simulink model "MultiAgentSEIRv1"  (R2019b)
settings: Solver=VariableStepAuto  StartTime=0.0  StopTime=365*2  FixedStep=1/24  RelTol=1e-12
libraries: SEIR_Lib x10
settings Model: Creator=Alex  LastModifiedBy=Alex

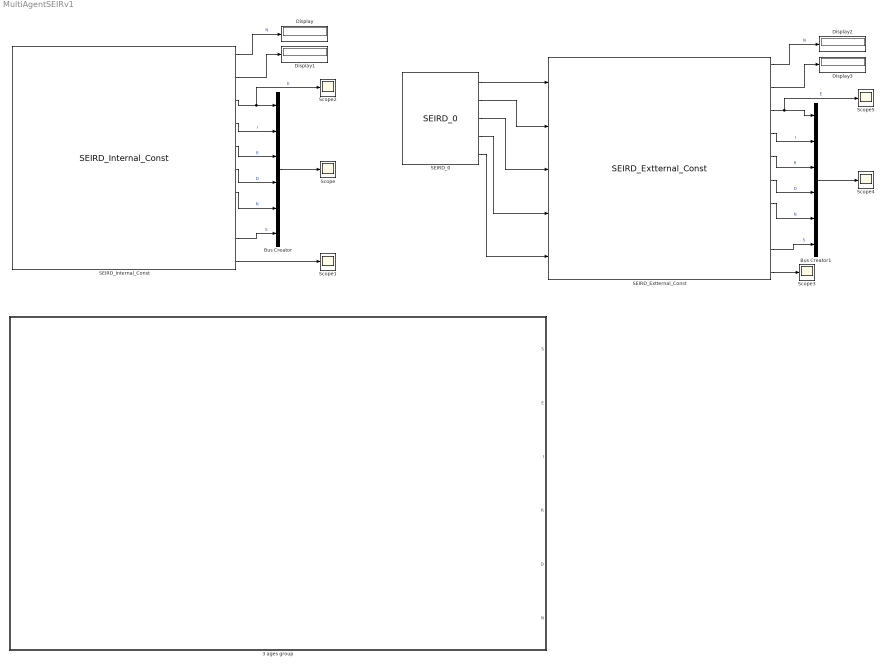
== system MultiAgentSEIRv1 ==
  3 ages group : Subsystem
  Bus Creator : BusCreator  Inputs=6
  Bus Creator1 : BusCreator  Inputs=6
  Display{,1..3} (4 alike) : Display
  SEIRD_0 : SEIR_Lib/SEIRD_0  SystemSampleTime=-1  Latency=0  AutoFrameSizeCalculation=off
  SEIRD_Extternal_Const : SEIR_Lib/SEIRD_Extternal_Const  SystemSampleTime=-1  Latency=0  AutoFrameSizeCalculation=off
      link override alpha1/Random NumberAlpha: Mean=0.1
  SEIRD_Internal_Const : SEIR_Lib/SEIRD_Internal_Const  SystemSampleTime=-1  Latency=0  AutoFrameSizeCalculation=off
      link override alpha1/Random NumberAlpha: Mean=0.1
  Scope{,1..5} (6 alike) : Scope
  wires:
  SEIRD_Internal_Const/3 -> Scope2/1, Bus Creator/1  "E"
  SEIRD_Internal_Const/4 -> Bus Creator/2  "I"
  SEIRD_Internal_Const/5 -> Bus Creator/3  "R"
  SEIRD_Internal_Const/6 -> Bus Creator/4  "D"
  SEIRD_Internal_Const/7 -> Bus Creator/5  "N"
  SEIRD_Internal_Const/9 -> Bus Creator/6  "S"
  Bus Creator/1 -> Scope/1
  SEIRD_Internal_Const/1 -> Display/1  "N"
  SEIRD_Internal_Const/2 -> Display1/1
  SEIRD_Internal_Const/10 -> Scope1/1
  SEIRD_0/1 -> SEIRD_Extternal_Const/1
  SEIRD_0/2 -> SEIRD_Extternal_Const/2
  SEIRD_0/3 -> SEIRD_Extternal_Const/3
  SEIRD_0/4 -> SEIRD_Extternal_Const/4
  SEIRD_0/5 -> SEIRD_Extternal_Const/5
  SEIRD_Extternal_Const/10 -> Scope3/1
  SEIRD_Extternal_Const/2 -> Display3/1
  SEIRD_Extternal_Const/1 -> Display2/1  "N"
  Bus Creator1/1 -> Scope4/1
  SEIRD_Extternal_Const/9 -> Bus Creator1/6  "S"
  SEIRD_Extternal_Const/7 -> Bus Creator1/5  "N"
  SEIRD_Extternal_Const/6 -> Bus Creator1/4  "D"
  SEIRD_Extternal_Const/5 -> Bus Creator1/3  "R"
  SEIRD_Extternal_Const/4 -> Bus Creator1/2  "I"
  SEIRD_Extternal_Const/3 -> Scope5/1, Bus Creator1/1  "E"

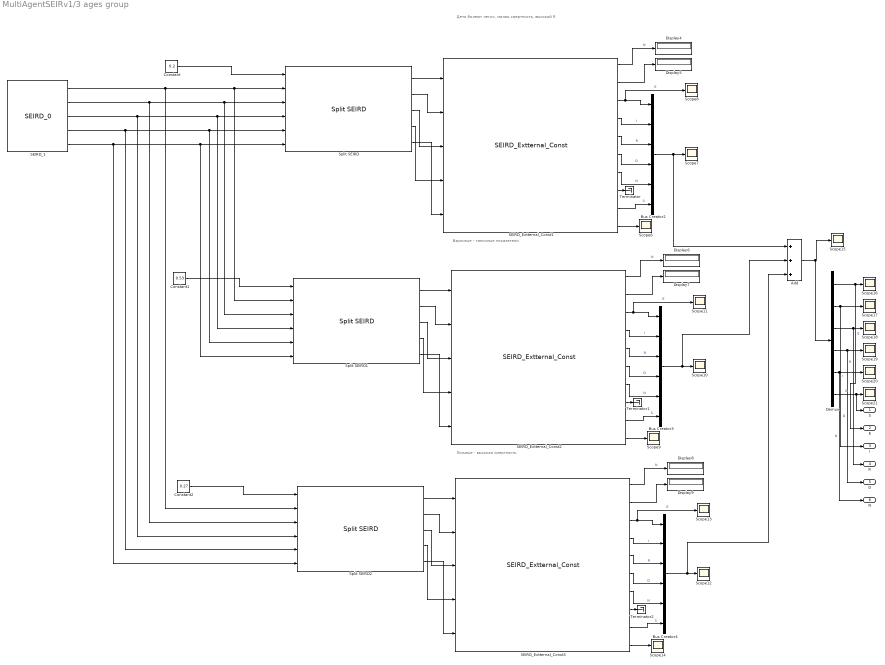
== system MultiAgentSEIRv1/3 ages group ==
  note: Пожиые - высокая смертность
  note: Взрослые - типичные показатели
  note: Дети болеют легко, малая смертность, высокий R
  Add : Sum  Inputs=+++
  Bus Creator2 : BusCreator  Inputs=6
  Bus Creator3 : BusCreator  Inputs=6
  Bus Creator4 : BusCreator  Inputs=6
  Constant : Constant  Value=0.2
  Constant1 : Constant  Value=0.53
  Constant2 : Constant  Value=0.27
  Demux : Demux  Outputs=6
  Display{4..9} (6 alike) : Display
  SEIRD_1 : SEIR_Lib/SEIRD_0  SystemSampleTime=-1  Latency=0  AutoFrameSizeCalculation=off
  SEIRD_Extternal_Const1 : SEIR_Lib/SEIRD_Extternal_Const  SystemSampleTime=-1  Latency=0  AutoFrameSizeCalculation=off
      link override Standart r_1: Value=3
      link override alpha1/Random NumberAlpha: Mean=0.1
  SEIRD_Extternal_Const2 : SEIR_Lib/SEIRD_Extternal_Const  SystemSampleTime=-1  Latency=0  AutoFrameSizeCalculation=off
      link override alpha1/Random NumberAlpha: Mean=0.1
  SEIRD_Extternal_Const3 : SEIR_Lib/SEIRD_Extternal_Const  SystemSampleTime=-1  Latency=0  AutoFrameSizeCalculation=off
      link override alpha1/Random NumberAlpha: Mean=1
  Scope{6..21} (16 alike) : Scope
  Split SEIRD : SEIR_Lib/Split SEIRD  SystemSampleTime=-1  Latency=0  AutoFrameSizeCalculation=off
  Split SEIRD1 : SEIR_Lib/Split SEIRD  SystemSampleTime=-1  Latency=0  AutoFrameSizeCalculation=off
  Split SEIRD2 : SEIR_Lib/Split SEIRD  SystemSampleTime=-1  Latency=0  AutoFrameSizeCalculation=off
  Terminator : Terminator
  Terminator1 : Terminator
  Terminator2 : Terminator
  S : Outport
  E : Outport  Port=2
  I : Outport  Port=3
  R : Outport  Port=4
  D : Outport  Port=5
  N : Outport  Port=6
  wires:
  Demux/4 -> Scope19/1, D/1  "D"
  SEIRD_Extternal_Const3/2 -> Display9/1
  Demux/3 -> R/1, Scope18/1  "R"
  SEIRD_1/5 -> Split SEIRD2/6, Split SEIRD1/6, Split SEIRD/6
  SEIRD_1/1 -> Split SEIRD2/2, Split SEIRD1/2, Split SEIRD/2
  SEIRD_Extternal_Const1/8 -> Terminator/1
  Bus Creator3/1 -> Add/2, Scope10/1
  SEIRD_Extternal_Const3/1 -> Display8/1  "N"
  SEIRD_Extternal_Const2/5 -> Bus Creator3/3  "R"
  SEIRD_Extternal_Const1/3 -> Scope8/1, Bus Creator2/1  "E"
  SEIRD_Extternal_Const3/7 -> Bus Creator4/5  "N"
  SEIRD_1/3 -> Split SEIRD2/4, Split SEIRD1/4, Split SEIRD/4
  SEIRD_Extternal_Const1/2 -> Display5/1
  Constant2/1 -> Split SEIRD2/1
  SEIRD_Extternal_Const3/3 -> Scope13/1, Bus Creator4/1  "E"
  Add/1 -> Demux/1, Scope15/1
  SEIRD_1/2 -> Split SEIRD2/3, Split SEIRD1/3, Split SEIRD/3
  Bus Creator4/1 -> Add/3, Scope12/1
  SEIRD_Extternal_Const2/2 -> Display7/1
  SEIRD_Extternal_Const1/4 -> Bus Creator2/2  "I"
  SEIRD_Extternal_Const3/4 -> Bus Creator4/2  "I"
  SEIRD_Extternal_Const1/5 -> Bus Creator2/3  "R"
  Bus Creator2/1 -> Add/1, Scope7/1
  Split SEIRD/3 -> SEIRD_Extternal_Const1/3
  SEIRD_Extternal_Const3/5 -> Bus Creator4/3  "R"
  Constant/1 -> Split SEIRD/1
  SEIRD_Extternal_Const3/6 -> Bus Creator4/4  "D"
  SEIRD_1/4 -> Split SEIRD2/5, Split SEIRD1/5, Split SEIRD/5
  SEIRD_Extternal_Const3/9 -> Bus Creator4/6  "S"
  Demux/6 -> S/1, Scope21/1  "S"
  SEIRD_Extternal_Const2/4 -> Bus Creator3/2  "I"
  SEIRD_Extternal_Const2/6 -> Bus Creator3/4  "D"
  Split SEIRD2/3 -> SEIRD_Extternal_Const3/3
  Split SEIRD2/2 -> SEIRD_Extternal_Const3/2
  SEIRD_Extternal_Const1/9 -> Bus Creator2/6  "S"
  SEIRD_Extternal_Const2/10 -> Scope9/1
  Split SEIRD2/4 -> SEIRD_Extternal_Const3/4
  Demux/1 -> E/1, Scope16/1  "E"
  Split SEIRD1/3 -> SEIRD_Extternal_Const2/3
  Split SEIRD2/1 -> SEIRD_Extternal_Const3/1
  Split SEIRD/1 -> SEIRD_Extternal_Const1/1
  SEIRD_Extternal_Const1/6 -> Bus Creator2/4  "D"
  Split SEIRD2/5 -> SEIRD_Extternal_Const3/5
  Split SEIRD1/2 -> SEIRD_Extternal_Const2/2
  SEIRD_Extternal_Const2/7 -> Bus Creator3/5  "N"
  SEIRD_Extternal_Const1/7 -> Bus Creator2/5  "N"
  Split SEIRD/5 -> SEIRD_Extternal_Const1/5
  Split SEIRD/2 -> SEIRD_Extternal_Const1/2
  Demux/2 -> I/1, Scope17/1  "I"
  SEIRD_Extternal_Const2/9 -> Bus Creator3/6  "S"
  SEIRD_Extternal_Const3/10 -> Scope14/1
  Constant1/1 -> Split SEIRD1/1
  SEIRD_Extternal_Const1/10 -> Scope6/1
  SEIRD_Extternal_Const2/1 -> Display6/1  "N"
  SEIRD_Extternal_Const1/1 -> Display4/1  "N"
  SEIRD_Extternal_Const2/3 -> Bus Creator3/1, Scope11/1  "E"
  Split SEIRD1/5 -> SEIRD_Extternal_Const2/5
  Split SEIRD1/1 -> SEIRD_Extternal_Const2/1
  Split SEIRD1/4 -> SEIRD_Extternal_Const2/4
  Demux/5 -> N/1, Scope20/1  "N"
  Split SEIRD/4 -> SEIRD_Extternal_Const1/4
  SEIRD_Extternal_Const2/8 -> Terminator1/1
  SEIRD_Extternal_Const3/8 -> Terminator2/1
